simulink model "GFLIB_Ramp_BAM"  (Simulink 9.3)
settings: Solver=VariableStepAuto  StartTime=0.0  StopTime=10.0  RelTol=1e-3
settings Model: Creator=nxa18952  LastModifiedBy=nxa18952
settings DataIOCC: SaveFormat=Dataset  SignalLoggingSaveFormat=Dataset  ReturnWorkspaceOutputs=on
settings OptimizationCC: LifeSpan=auto
settings DebuggingCC: UnderspecifiedInitializationDetection=Simplified  MergeDetectMultiDrivingBlocksExec=error  FcnCallInpInsideContextMsg=error  SFUnexpectedBacktrackingDiag=error  SFNoUnconditionalDefaultTransitionDiag=error  SFExecutionAtInitializationDiag=warning  ArithmeticOperatorsInVariantConditions=error
settings HardwareCC: ProdBitPerPointer=64  ProdBitPerSizeT=64  ProdBitPerPtrDiffT=64  ProdLargestAtomicFloat=Float  ProdIntDivRoundTo=Zero  ProdEndianess=LittleEndian  ProdWordSize=64  ProdHWDeviceType=Intel->x86-64 (Windows64)
settings ModelReferenceCC: PropagateSignalLabelsOutOfModel=on
settings SFSimCC: SimUseLocalCustomCode=on
settings RTWCC: RTWUseLocalCustomCode=on
settings CodeAppCC: StateflowObjectComments=off
settings GRTTargetCC: TargetLangStandard=C99 (ISO)  CombineOutputUpdateFcns=on  GRTInterface=off
settings ConfigComp: CovMetricSettings=dwe  CovHtmlReporting=off  CovSaveCumulativeToWorkspaceVar=off  CovSaveSingleToWorkspaceVar=off  CovExternalEMLEnable=on

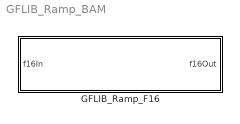
== system GFLIB_Ramp_BAM ==
  GFLIB_Ramp_F16 : Subsystem  TreatAsAtomicUnit=on  mask(GFLIB_Ramp_F16){showStates=Hide (faster execution), f16RampUp=0, f16RampDown=0}
      mask prompts: showStates "Show internal states"; f16RampUp "f16RampUp (Ramp up increment coefficient)"; f16RampDown "f16RampDown (Ramp decrement coefficient)"
      mask help: Rate of change limiter - ramp function in 16-bit fixed-point fractional implementation. Refer to the AMMCLIB User's Guide for further details.
      mask init:
      | if ~evalin('base','exist(''tS8'',''var'')')
      |   if (2 ~= exist('SWLIBS_Typedefs.mat','file'))
      |       error('File SWLIBS_Typedefs.mat is not on the Matlab path. Please add the AMMCLIB "bam" folder in the Matlab Search Path.');
      |   else
      |       evalin('base', 'load(''SWLIBS_Typedefs.mat'')');
      |   end
      | end
      | if showStates == 1
      |     % hidden state variables
      |     if strcmp(get_param([gcb '/f16State'], 'BlockType'), 'Inport')
      |         posblk = get_param(gcb, 'Position');
      | 
      |         pos = get_param(    [gcb, '/f16State'], 'Position');
      |         orient = get_param( [gcb, '/f16State'], 'Orientation');
      |         delete_block(       [gcb, '/f16State']);
      |         add_block('built-in/Ground', [gcb, '/f16State'], 'Position', pos, 'Orientation', orient);
      | 
      |         pos = get_param(    [gcb, '/f16RampUp'], 'Position');
      |         orient = get_param( [gcb, '/f16RampUp'], 'Orientation');
      |         delete_block(       [gcb, '/f16RampUp']);
      |         add_block('built-in/Ground', [gcb, '/f16RampUp'], 'Position', pos, 'Orientation', orient);
      | 
      |         pos = get_param(    [gcb, '/f16RampDown'], 'Position');
      |         orient = get_param( [gcb, '/f16RampDown'], 'Orientation');
      |         delete_block(       [gcb, '/f16RampDown']);
      |         add_block('built-in/Ground', [gcb, '/f16RampDown'], 'Position', pos, 'Orientation', orient);
      | 
      | 
      |         pos = get_param(    [gcb '/f16State_Out'], 'Position');
      |         orient = get_param( [gcb '/f16State_Out'], 'Orientation');
      |         delete_block(       [gcb '/f16State_Out']);
      |         add_block('built-in/Terminator', [gcb '/f16State_Out'], 'Position', pos, 'Orientation', orient);
      | 
      | 
      |         set_param([gcb '/f16In'], 'Port', '1');
      | 
      |         set_param([gcb '/f16Out'], 'Port', '1');
      | 
      |         set_param(gcb,'MaskEnables',{'on','on','on'});
      | 
      |         if (posblk(4) - posblk(2)) > 50
      |           height = 50;
      |           set_param(gcb,'Position',[posblk(1), posblk(2), posblk(3), posblk(2)+height])
      |         end
      |     end
      | else
      |     % shown state variables
      |     if strcmp(get_param([gcb '/f16State'], 'BlockType'), 'Ground')
      |         posblk = get_param(gcb, 'Position');
      | 
      |         pos = get_param(    [gcb, '/f16State'], 'Position');
      |         orient = get_param( [gcb, '/f16State'], 'Orientation');
      |         delete_block(       [gcb, '/f16State']);
      |         add_block('built-in/Inport', [gcb, '/f16State'], 'Position', pos, 'Orientation', orient, 'OutDataTypeStr', 'int16');
      | 
      |         pos = get_param(    [gcb, '/f16RampUp'], 'Position');
      |         orient = get_param( [gcb, '/f16RampUp'], 'Orientation');
      |         delete_block(       [gcb, '/f16RampUp']);
      |         add_block('built-in/Inport', [gcb, '/f16RampUp'], 'Position', pos, 'Orientation', orient, 'OutDataTypeStr', 'int16');
      | 
      |         pos = get_param(    [gcb, '/f16RampDown'], 'Position');
      |         orient = get_param( [gcb, '/f16RampDown'], 'Orientation');
      |         delete_block(       [gcb, '/f16RampDown']);
      |         add_block('built-in/Inport', [gcb, '/f16RampDown'], 'Position', pos, 'Orientation', orient, 'OutDataTypeStr', 'int16');
      | 
      | 
      |         pos = get_param(    [gcb '/f16State_Out'], 'Position');
      |         orient = get_param( [gcb '/f16State_Out'], 'Orientation');
      |         delete_block(       [gcb '/f16State_Out']);
      |         add_block('built-in/Outport', [gcb '/f16State_Out'], 'Position', pos, 'Orientation', orient);
      | 
      | 
      |         set_param([gcb '/f16In'], 'Port', '1');
      |         set_param([gcb '/f16State'], 'Port', '2');
      |         set_param([gcb '/f16RampUp'], 'Port', '3');
      |         set_param([gcb '/f16RampDown'], 'Port', '4');
      | 
      |         set_param([gcb '/f16Out'], 'Port', '1');
      |         set_param([gcb '/f16State_Out'], 'Port', '2');
      | 
      |         set_param(gcb,'MaskEnables',{'on','off','off'});
      | 
      |         if (posblk(4) - posblk(2)) < 125
      |           height = 125;
      |           set_param(gcb,'Position',[posblk(1), posblk(2), posblk(3), posblk(2)+height])
      |         end
      |     end
      | end
      settings: RTWSystemCode=Inline
      mask TypeOptions showStates: Hide (faster execution) | Show (allows debugging; connect feedback loops manually)
      mask Callback showStates:
      | maskStr = get_param(gcb,'showStates');
      | if strcmp(maskStr,'Hide (faster execution)'),
      |     set_param(gcb,'MaskEnables',{'on','on','on'});
      | else
      |     set_param(gcb,'MaskEnables',{'on','off','off'});
      | end
      mask Display:
      | color('black');
      | pos = get_param(gcb, 'Position');
      | width = pos(3) - pos(1);
      | height = pos(4) - pos(2);
      | tX=width/2;
      | tY=height - 8;
      | color('black');
      | text(tX,tY, 'GFLIB_Ramp_F16', 'horizontalAlignment', 'center');
      | if showStates == 2
      |   color('red');
      |   text(tX,tY - 20, ['debugging mode' char(13) char(10) '(limited performance)'], 'horizontalAlignment', 'center');
      | end

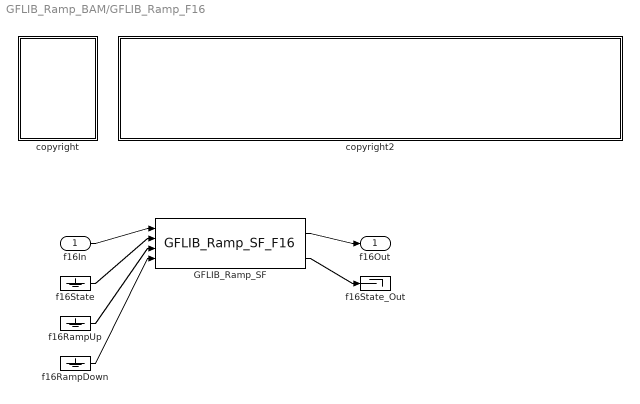
== system GFLIB_Ramp_BAM/GFLIB_Ramp_F16 ==
  f16In : Inport  OutDataTypeStr=int16
  GFLIB_Ramp_SF : S-Function  FunctionName=GFLIB_Ramp_SF_F16  Parameters=showStates,f16RampUp,f16RampDown  SFunctionDeploymentMode=off  EnableBusSupport=off
  copyright : Subsystem
      mask Display: text(10,90,'FILE:');text(10,75,'DESRIPTION:');text(10,60,'COPYRIGHT:');text(10,45,'VERSION:');text(10,30,'DATE:')
  copyright2 : Subsystem
      mask Display: text(10,90,'GFLIB_Ramp_BAM_F16.mdl');text(10,75,'Rate of change limiter - ramp function.');text(10,60,'NXP 2020');text(10,45,'1.0');text(10,30,'18-Mar-2020');
  f16RampDown : Ground
  f16RampUp : Ground
  f16State : Ground
  f16State_Out : Terminator
  f16Out : Outport
  wires:
  f16In/1 -> GFLIB_Ramp_SF/1
  f16State/1 -> GFLIB_Ramp_SF/2
  f16RampUp/1 -> GFLIB_Ramp_SF/3
  f16RampDown/1 -> GFLIB_Ramp_SF/4
  GFLIB_Ramp_SF/1 -> f16Out/1
  GFLIB_Ramp_SF/2 -> f16State_Out/1

== system GFLIB_Ramp_BAM/GFLIB_Ramp_F16/copyright ==

== system GFLIB_Ramp_BAM/GFLIB_Ramp_F16/copyright2 ==
